simulink model "Controller"  (R2025a)
settings: Solver=FixedStepAuto  StartTime=0.0  StopTime=0.5  FixedStep=1e-6  RelTol=1e-3
undefined symbols (not defined in the file): Bit_1, Bit_2, Bit_3, Bit_4, Bit_5, Bit_6, Bit_7, Bit_8
libraries: simulink_extras x42, fl_lib x33, nesl_utility x17, simulink x4, dspsigops x2
(part 1 of 3)
settings Model: PacingRate=0.002500  Creator=Erys  LastModifiedBy=Erys
settings SolverCC: AllowMultiTaskInputOutput=on

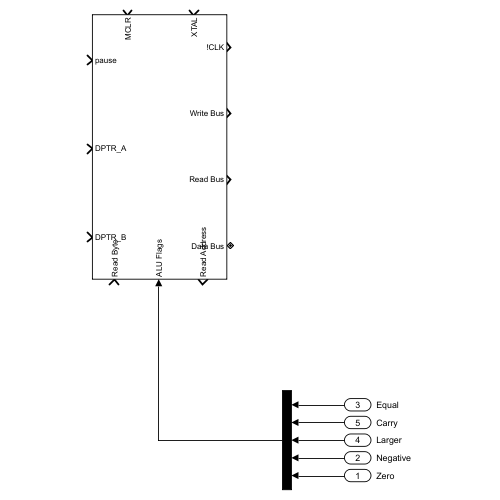
[thumbnail: Simulink's stored preview of the top-level diagram]
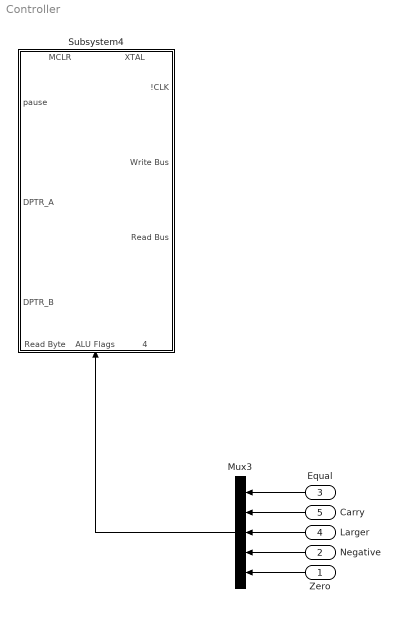
== system Controller ==
  Zero : Inport
  Negative : Inport  Port=2
  Equal : Inport  Port=3
  Larger : Inport  Port=4
  Carry : Inport  Port=5
  Mux3 : Mux  Inputs=5
  Subsystem4 : Subsystem
      settings: PortSchema="{\"entries\":[{\"content\":{\"sides\":[{\"content\":{\"connectorIds\":[\"In1\",\"In2\",\"In3\"]},\"type\":\"ConnectorPlacement.EquallySpacedRectSide\",\"uuid\":\"d5e2a106-9af6-429b-a75d-9517a76ca7ea\"},{\"content\":{\"connectorIds\":[\"Out1\",\"Out2\",\"Out3\",\"RConn1\"],\"side\":\"RIGHT\"},\"type\":\"ConnectorPlacement.EquallySpacedRectSide\",\"uuid\":\"6877b27f-1be8-45b2-a02e-770da90fb244\"},{\"content\":{\"connectorIds\":[\"In4\",\"In5\"],\"side\":\"TOP\"},\"type\":\"ConnectorPlacement.EquallySpacedRectSide\",\"uuid\":\"b2c1f94a-cab7-4390-a39c-f82c22ddd5ce\"},{\"content\":{\"connectorIds\":[\"In6\",\"In7\",\"Out4\"],\"side\":\"BOTTOM\"},\"type\":\"ConnectorPlacement.EquallySpacedRectSide\",\"uuid\":\"902a6980-cbbd-4700-8659-46292e270521\"}]},\"type\":\"ConnectorPlacement.EquallySpacedConnector\",\"uuid\":\"c8caef69-ab90-47f5-9596-0f6f8fcd412d\"}],\"packageUris\":[\"http://schema.mathworks.com/mf0/Connector/R2020b\"],\"version\":\"1.0\"}"
  wires:
  Larger/1 -> Mux3/3
  Zero/1 -> Mux3/5
  Negative/1 -> Mux3/4
  Equal/1 -> Mux3/1
  Carry/1 -> Mux3/2
  Mux3/1 -> Subsystem4/7(ALU Flags)

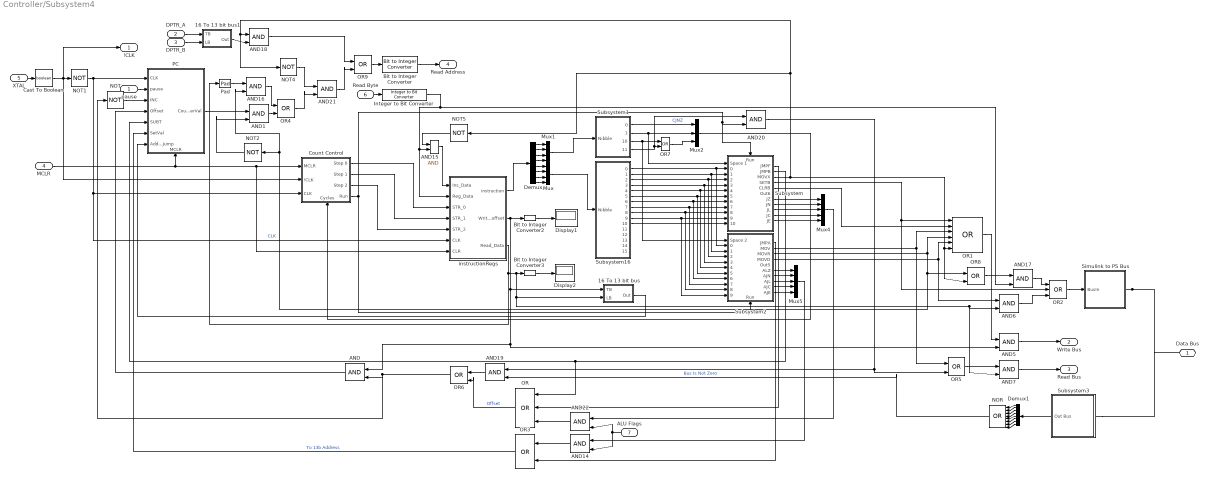
== system Controller/Subsystem4 ==
  pause : Inport
  DPTR_A : Inport  Port=2
  DPTR_B : Inport  Port=3
  MCLR : Inport  Port=4
  XTAL : Inport  Port=5
  Read Byte : Inport  Port=6
  ALU Flags : Inport  Port=7
  16 To 13 bit bus : Subsystem
  16 To 13 bit bus1 : Subsystem
  AND{,1,5..7,14..22} (14 alike) : Logic  IconShape=distinctive  AllPortsSameDT=off  OutDataTypeStr=boolean
  Bit to Integer Converter : simulink/Logic and Bit Operations/Bit to Integer Converter  nbits=13  bitOrder=MSB first  signedOutputValues=Unsigned  outDtype=Inherit via internal rule  outDtypeSigned=Inherit via internal rule
  Bit to Integer Converter2 : simulink/Logic and Bit Operations/Bit to Integer Converter  nbits=8  bitOrder=MSB first  signedOutputValues=Unsigned  outDtype=Inherit via internal rule  outDtypeSigned=Inherit via internal rule
  Bit to Integer Converter3 : simulink/Logic and Bit Operations/Bit to Integer Converter  nbits=8  bitOrder=MSB first  signedOutputValues=Unsigned  outDtype=Inherit via internal rule  outDtypeSigned=Inherit via internal rule
  Cast To Boolean : DataTypeConversion  OutDataTypeStr=boolean  SaturateOnIntegerOverflow=off  RndMeth=Floor
  Count Control : Subsystem
      settings: PortSchema="{\"entries\":[{\"content\":{\"sides\":[{\"content\":{\"connectorIds\":[\"In1\",\"In2\",\"In3\"]},\"type\":\"ConnectorPlacement.EquallySpacedRectSide\",\"uuid\":\"2946c837-3e9e-4d6d-a79b-eeee00653dec\"},{\"content\":{\"connectorIds\":[\"Out1\",\"Out2\",\"Out3\",\"Out4\"],\"side\":\"RIGHT\"},\"type\":\"ConnectorPlacement.EquallySpacedRectSide\",\"uuid\":\"31741f8e-3a86-46f4-9b5c-128a6668da37\"},{\"content\":{\"side\":\"TOP\"},\"type\":\"ConnectorPlacement.EquallySpacedRectSide\",\"uuid\":\"d0cf1acd-e26c-4fb6-8ea6-e97418659fa2\"},{\"content\":{\"connectorIds\":[\"In4\"],\"side\":\"BOTTOM\"},\"type\":\"ConnectorPlacement.EquallySpacedRectSide\",\"uuid\":\"e969e3c0-96c1-4acf-855c-d1f83bd67524\"}]},\"type\":\"ConnectorPlacement.EquallySpacedConnector\",\"uuid\":\"6217865d-f245-4d28-aa10-c01e5d783290\"}],\"packageUris\":[\"http://schema.mathworks.com/mf0/Connector/R2020b\"],\"version\":\"1.0\"}"
  Demux : Demux  Outputs=8
  Demux1 : Demux  Outputs=8
  Display1 : Display
  Display2 : Display
  Integer to Bit Converter : simulink/Logic and Bit Operations/Integer to Bit Converter  nbits=8  signedInputValues=Unsigned  bitOrder=MSB first  outDtype=Inherit via internal rule
  Mux : Mux
  Mux1 : Mux
  Mux2 : Mux  Inputs=3
  Mux4 : Mux  Inputs=5
  Mux5 : Mux  Inputs=5
  NOR : Logic  Operator=OR  Inputs=8  IconShape=distinctive  AllPortsSameDT=off  OutDataTypeStr=boolean
  NOT{,1..2,4..5} (5 alike) : Logic  Operator=NOT  IconShape=distinctive  AllPortsSameDT=off  OutDataTypeStr=boolean
  OR : Logic  Operator=OR  Inputs=3  IconShape=distinctive  AllPortsSameDT=off  OutDataTypeStr=boolean
  OR1 : Logic  Operator=OR  Inputs=6  IconShape=distinctive  AllPortsSameDT=off  OutDataTypeStr=boolean
  OR2 : Logic  Operator=OR  Inputs=3  IconShape=distinctive  AllPortsSameDT=off  OutDataTypeStr=boolean
  OR{3..9} (7 alike) : Logic  Operator=OR  IconShape=distinctive  AllPortsSameDT=off  OutDataTypeStr=boolean
  PC : Subsystem
      settings: PortSchema="{\"entries\":[{\"content\":{\"sides\":[{\"content\":{\"connectorIds\":[\"In1\",\"In2\",\"In3\",\"In4\",\"In5\",\"In6\",\"In7\"]},\"type\":\"ConnectorPlacement.EquallySpacedRectSide\",\"uuid\":\"447360f6-a9ef-4a9c-a715-cde64203432e\"},{\"content\":{\"connectorIds\":[\"Out1\"],\"side\":\"RIGHT\"},\"type\":\"ConnectorPlacement.EquallySpacedRectSide\",\"uuid\":\"8baf234e-02d5-44b8-81cb-8a80707fc347\"},{\"content\":{\"side\":\"TOP\"},\"type\":\"ConnectorPlacement.EquallySpacedRectSide\",\"uuid\":\"5f74c121-ef0f-4272-a153-104d7b2f50e7\"},{\"content\":{\"connectorIds\":[\"In8\"],\"side\":\"BOTTOM\"},\"type\":\"ConnectorPlacement.EquallySpacedRectSide\",\"uuid\":\"1b724eb9-c90a-41ee-9e1f-a1aa86a34cfc\"}]},\"type\":\"ConnectorPlacement.EquallySpacedConnector\",\"uuid\":\"abd2f1ff-4bc7-462e-9088-dc740170a27d\"}],\"packageUris\":[\"http://schema.mathworks.com/mf0/Connector/R2020b\"],\"version\":\"1.0\"}"
  Pad : dspsigops/Pad  padAlong=Columns  dimsToPad=1  valSrc=Specify via dialog  padVal=0  spec=Output size  padNumOutRowsSpecMethod=User-specified  numOutRows=13  padNumOutColsSpecMethod=User-specified  numOutCols=1  isVarDimsMode=off  padBeginning=0  padEnd=0  outSizeMode=User-specified  outSize=1  padSigAt=Beginning  trunc_flag=None  roundingMode=Floor  overflowMode=off  truncOrWrapMode=Truncate  wrap_flag=None
  Simulink to PS Bus : Subsystem
  Subsystem : Subsystem
      settings: PortSchema="{\"entries\":[{\"content\":{\"sides\":[{\"content\":{\"connectorIds\":[\"In1\",\"In2\",\"In3\",\"In4\",\"In5\",\"In6\",\"In7\",\"In8\",\"In9\",\"In10\",\"In11\",\"In12\"]},\"type\":\"ConnectorPlacement.EquallySpacedRectSide\",\"uuid\":\"cfbb32f0-f26b-4c66-8bd2-b70029f88bb0\"},{\"content\":{\"connectorIds\":[\"Out1\",\"Out2\",\"Out3\",\"Out4\",\"Out5\",\"Out6\",\"Out7\",\"Out8\",\"Out9\",\"Out10\",\"Out11\"],\"side\":\"RIGHT\"},\"type\":\"ConnectorPlacement.EquallySpacedRectSide\",\"uuid\":\"98f5ba87-6b95-4dd6-a355-88798db6b2fd\"},{\"content\":{\"connectorIds\":[\"In13\"],\"side\":\"TOP\"},\"type\":\"ConnectorPlacement.EquallySpacedRectSide\",\"uuid\":\"0d46a759-70c5-4c59-bf81-538ef6837c1f\"}]},\"type\":\"ConnectorPlacement.EquallySpacedConnector\",\"uuid\":\"e16d022d-bc87-42d5-a95e-dac1e9efe00b\"}],\"packageUris\":[\"http://schema.mathworks.com/mf0/Connector/R2020b\"],\"version\":\"1.0\"}"
  Subsystem1 : Subsystem
  Subsystem16 : Subsystem
  Subsystem2 : Subsystem
      settings: PortSchema="{\"entries\":[{\"content\":{\"sides\":[{\"content\":{\"connectorIds\":[\"In1\",\"In2\",\"In3\",\"In4\",\"In5\",\"In6\",\"In7\",\"In8\",\"In9\",\"In10\",\"In11\"]},\"type\":\"ConnectorPlacement.EquallySpacedRectSide\",\"uuid\":\"b0b83ebf-b15c-48e6-90da-0c85466b0112\"},{\"content\":{\"connectorIds\":[\"Out1\",\"Out2\",\"Out3\",\"Out4\",\"Out5\",\"Out6\",\"Out7\",\"Out8\",\"Out9\",\"Out10\"],\"side\":\"RIGHT\"},\"type\":\"ConnectorPlacement.EquallySpacedRectSide\",\"uuid\":\"3e9a574c-c2fc-44d4-b6d6-2fd6d79cf320\"},{\"content\":{\"side\":\"TOP\"},\"type\":\"ConnectorPlacement.EquallySpacedRectSide\",\"uuid\":\"d0111dce-9a98-4fcc-8b1f-a07207ba465c\"},{\"content\":{\"connectorIds\":[\"In12\"],\"side\":\"BOTTOM\"},\"type\":\"ConnectorPlacement.EquallySpacedRectSide\",\"uuid\":\"f4ec0d33-710b-4536-80bf-b2ccdd599d6b\"}]},\"type\":\"ConnectorPlacement.EquallySpacedConnector\",\"uuid\":\"77566f56-f460-4ec7-92f0-67352915e372\"}],\"packageUris\":[\"http://schema.mathworks.com/mf0/Connector/R2020b\"],\"version\":\"1.0\"}"
  Subsystem3 : Subsystem
  instructionRegs : Subsystem
  Data Bus : PMIOPort  Side=Right
  !CLK : Outport
  Write Bus : Outport  Port=2
  Read Bus : Outport  Port=3
  Read Address : Outport  Port=4
  wires:
  NOT/1 -> PC/3(INC)
  Mux/1 -> Subsystem16/1(Nibble)
  Subsystem/7(JZ) -> Mux4/1
  Subsystem/8(JN) -> Mux4/2
  Subsystem2/4(MOVD) -> AND6/1, OR1/5
  Subsystem2/1(JMPA) -> OR3/2
  MCLR/1 -> Count Control/1(MCLR), instructionRegs/7(CLR), PC/8(MCLR)
  Subsystem16/7(6) -> Subsystem2/8(6), Subsystem/8(6)
  Subsystem2/3(MOVR) -> AND16/2, NOT2/1, OR8/1, OR1/4
  Subsystem16/1(0) -> Subsystem/2(0), Subsystem2/2(0)
  Mux2/1 -> Count Control/4(Cycles)
  Subsystem16/8(7) -> Subsystem2/9(7), Subsystem/9(7)
  OR4/1 -> AND21/2
  AND5/1 -> Write Bus/1
  Subsystem/9(JL) -> Mux4/3
  Bit to Integer Converter3/1 -> Display2/1
  Demux/4 -> Mux1/4
  Subsystem16/4(3) -> Subsystem2/5(3), Subsystem/5(3)
  Subsystem/2(JMPB) -> OR/1, PC/5(SUBT)
  Subsystem/1(JMPF) -> OR/2
  Subsystem16/10(9) -> Subsystem2/11(9), Subsystem/11(9)
  Subsystem16/3(2) -> Subsystem2/4(2), Subsystem/4(2)
  OR/1 -> OR6/2  "Offset"
  AND7/1 -> Read Bus/1
  Subsystem/4(SETB) -> OR2/2, OR1/1
  Count Control/4(Run) -> AND20/2, Subsystem/13(Run), Subsystem2/12(Run)
  AND17/1 -> OR2/1
  Demux/6 -> Mux/2
  Demux/8 -> Mux/4
  Bit to Integer Converter2/1 -> Display1/1
  OR2/1 -> Simulink to PS Bus/1(BusIn)
  Demux/7 -> Mux/3
  Cast To Boolean/1 -> !CLK/1, Count Control/2(!CLK), NOT1/1
  Demux/3 -> Mux1/3
  Read Byte/1 -> Integer to Bit Converter/1
  Mux1/1 -> Subsystem1/1(Nibble)
  Subsystem16/9(8) -> Subsystem2/10(8), Subsystem/10(8)
  Subsystem16/6(5) -> Subsystem2/7(5), Subsystem/7(5)
  Bit to Integer Converter/1 -> Read Address/1
  Subsystem16/2(1) -> Subsystem/3(1), Subsystem2/3(1)
  Subsystem1/1(0) -> Mux2/1
  Subsystem2/2(MOV) -> OR5/1, OR1/3
  NOT1/1 -> instructionRegs/6(CLK), Count Control/3(CLK), PC/1(CLK)  "CLK"
  Integer to Bit Converter/1 -> instructionRegs/2(Reg_Data), AND15/2, AND17/2
  XTAL/1 -> Cast To Boolean/1
  AND16/1 -> OR4/1
  AND/1 -> PC/4(Offset)
  Subsystem16/11(10) -> Subsystem/12(10)
  Subsystem1/2(1) -> Mux2/2, Subsystem/1(Space 1)
  Subsystem/5(CLRB) -> OR1/2
  Demux/2 -> Mux1/2
  Demux/1 -> Mux1/1
  Subsystem16/5(4) -> Subsystem2/6(4), Subsystem/6(4)
  Subsystem1/3(10) -> OR7/1, Subsystem2/1(Space 2)
  OR1/1 -> AND5/1
  Demux/5 -> Mux/1
  OR5/1 -> AND7/1
  NOR/1 -> AND19/2  "Bus Is Not Zero"
  OR3/1 -> PC/6(SetVal)  "To 13b Address"
  PC/1(CounterVal) -> AND1/1
  AND1/1 -> OR4/2
  16 To 13 bit bus/1(Out) -> PC/7(AddressJump)
  Subsystem/10(JC) -> Mux4/4
  Demux1/2 -> NOR/2
  Subsystem/11(JE) -> Mux4/5
  Demux1/1 -> NOR/1
  AND14/1 -> OR3/1
  AND6/1 -> OR2/3
  NOT2/1 -> AND1/2
  Demux1/3 -> NOR/3
  Demux1/4 -> NOR/4
  Demux1/5 -> NOR/5
  Demux1/7 -> NOR/7
  Demux1/8 -> NOR/8
  Demux1/6 -> NOR/6
  Subsystem/3(MOVX) -> NOT5/1, NOT4/1, AND18/1, OR1/6, OR8/2
  pause/1 -> PC/2(pause)
  Subsystem1/4(11) -> AND20/1, OR7/2  "CJNZ"
  OR7/1 -> Mux2/3
  AND20/1 -> AND19/1, OR5/2
  OR6/1 -> NOT/1, AND/2
  AND19/1 -> OR6/1
  Subsystem3/1(Out Bus) -> Demux1/1
  16 To 13 bit bus1/1(Out) -> AND18/2
  DPTR_B/1 -> 16 To 13 bit bus1/2(LB)
  DPTR_A/1 -> 16 To 13 bit bus1/1(TB)
  Pad/1 -> AND16/1
  OR8/1 -> AND17/1
  NOT4/1 -> AND21/1
  AND21/1 -> OR9/2
  AND18/1 -> OR9/1
  OR9/1 -> Bit to Integer Converter/1
  NOT5/1 -> AND15/1
  instructionRegs/2(Write_offset) -> 16 To 13 bit bus/1(TB), AND/1, AND5/2, Bit to Integer Converter2/1
  instructionRegs/3(Read_Data) -> AND7/2, AND6/2, 16 To 13 bit bus/2(LB), Bit to Integer Converter3/1, Pad/1
  instructionRegs/1(instruction) -> Demux/1
  AND15/1 -> instructionRegs/1(Ins_Data)
  Count Control/1(Step 0) -> instructionRegs/3(STR_0)
  Count Control/2(Step 1) -> instructionRegs/4(STR_1)
  Count Control/3(Step 2) -> instructionRegs/5(STR_2)
  ALU Flags/1 -> AND22/2, AND14/2
  Mux4/1 -> AND22/1
  AND22/1 -> OR/3
  Subsystem2/10(AJE) -> Mux5/5
  Subsystem2/9(AJC) -> Mux5/4
  Subsystem2/8(AJL) -> Mux5/3
  Subsystem2/7(AJN) -> Mux5/2
  Subsystem2/6(ALZ) -> Mux5/1
  Mux5/1 -> AND14/1
  connections:
  Simulink to PS Bus/RConn1 -- Subsystem3/LConn1 -- Data Bus/RConn1

== system Controller/Subsystem4/16 To 13 bit bus ==
  TB : Inport
  LB : Inport  Port=2
  Demux1 : Demux  Outputs=8
  Demux2 : Demux  Outputs=8
  Mux2 : Mux  Inputs=13
  Out : Outport
  wires:
  Demux2/5 -> Mux2/10
  Demux1/8 -> Mux2/5
  Demux2/1 -> Mux2/6
  Demux1/5 -> Mux2/2
  Demux2/6 -> Mux2/11
  Demux1/6 -> Mux2/3
  Demux1/7 -> Mux2/4
  Demux2/2 -> Mux2/7
  Demux2/3 -> Mux2/8
  Demux1/4 -> Mux2/1
  Demux2/8 -> Mux2/13
  Demux2/7 -> Mux2/12
  Demux2/4 -> Mux2/9
  TB/1 -> Demux1/1
  Mux2/1 -> Out/1
  LB/1 -> Demux2/1

== system Controller/Subsystem4/16 To 13 bit bus1 ==
  TB : Inport
  LB : Inport  Port=2
  Demux1 : Demux  Outputs=8
  Demux2 : Demux  Outputs=8
  Mux2 : Mux  Inputs=13
  Out : Outport
  wires:
  Demux2/5 -> Mux2/10
  Demux1/8 -> Mux2/5
  Demux2/1 -> Mux2/6
  Demux1/5 -> Mux2/2
  Demux2/6 -> Mux2/11
  Demux1/6 -> Mux2/3
  Demux1/7 -> Mux2/4
  Demux2/2 -> Mux2/7
  Demux2/3 -> Mux2/8
  Demux1/4 -> Mux2/1
  Demux2/8 -> Mux2/13
  Demux2/7 -> Mux2/12
  Demux2/4 -> Mux2/9
  TB/1 -> Demux1/1
  Mux2/1 -> Out/1
  LB/1 -> Demux2/1

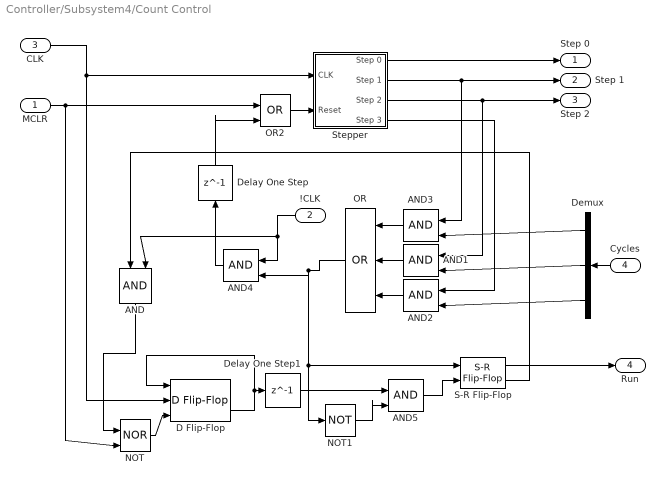
== system Controller/Subsystem4/Count Control ==
  MCLR : Inport
  !CLK : Inport  Port=2
  CLK : Inport  Port=3
  Cycles : Inport  Port=4
  AND{,1..5} (6 alike) : Logic  IconShape=distinctive  AllPortsSameDT=off  OutDataTypeStr=boolean
  D Flip-Flop : simulink_extras/Flip Flops/D Flip-Flop
  Delay One Step : Delay  DelayLength=1
  Delay One Step1 : Delay  DelayLength=1
  Demux : Demux  Outputs=3
  NOT : Logic  Operator=NOR  IconShape=distinctive  AllPortsSameDT=off  OutDataTypeStr=boolean
  NOT1 : Logic  Operator=NOT  IconShape=distinctive  AllPortsSameDT=off  OutDataTypeStr=boolean
  OR : Logic  Operator=OR  Inputs=3  IconShape=distinctive  AllPortsSameDT=off  OutDataTypeStr=boolean
  OR2 : Logic  Operator=OR  IconShape=distinctive  AllPortsSameDT=off  OutDataTypeStr=boolean
  S-R Flip-Flop : simulink_extras/Flip Flops/S-R Flip-Flop  initial_condition=0
  Stepper : Subsystem
  Step 0 : Outport
  Step 1 : Outport  Port=2
  Step 2 : Outport  Port=3
  Run : Outport  Port=4
  wires:
  NOT/1 -> D Flip-Flop/3
  CLK/1 -> D Flip-Flop/2, Stepper/1(CLK)
  Stepper/2(Step 1) -> Step 1/1, AND3/1
  Stepper/1(Step 0) -> Step 0/1
  AND2/1 -> OR/3
  D Flip-Flop/2 -> Delay One Step1/1, D Flip-Flop/1
  AND1/1 -> OR/2
  AND3/1 -> OR/1
  Delay One Step/1 -> OR2/2
  !CLK/1 -> AND4/1, AND/2
  AND4/1 -> Delay One Step/1
  Stepper/3(Step 2) -> Step 2/1, AND1/1
  OR/1 -> S-R Flip-Flop/1, NOT1/1, AND4/2
  OR2/1 -> Stepper/2(Reset)
  Stepper/4(Step 3) -> AND2/1
  Demux/1 -> AND3/2
  Demux/2 -> AND1/2
  Demux/3 -> AND2/2
  Cycles/1 -> Demux/1
  MCLR/1 -> NOT/2, OR2/1
  S-R Flip-Flop/1 -> Run/1
  AND5/1 -> S-R Flip-Flop/2
  NOT1/1 -> AND5/2
  AND/1 -> NOT/1
  S-R Flip-Flop/2 -> AND/1
  Delay One Step1/1 -> AND5/1

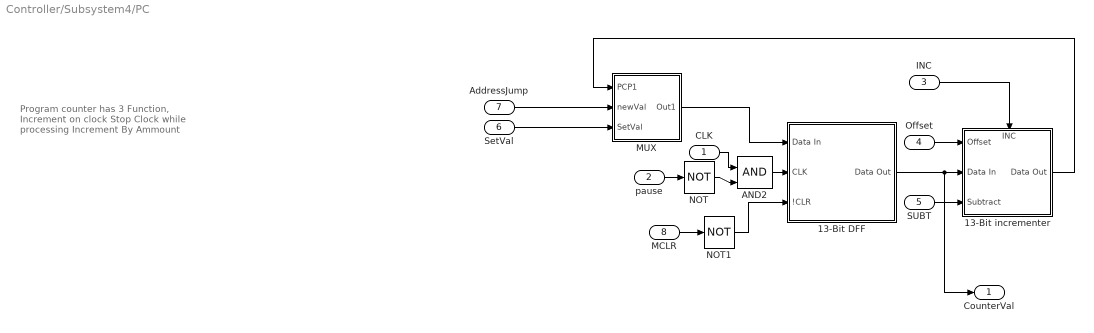
== system Controller/Subsystem4/PC ==
  note: Program counter has 3 Function,
      |
      | Increment on clock
      | Stop Clock while processing
      | Increment By Ammount
  CLK : Inport
  pause : Inport  Port=2
  INC : Inport  Port=3
  Offset : Inport  Port=4
  SUBT : Inport  Port=5
  SetVal : Inport  Port=6
  AddressJump : Inport  Port=7
  MCLR : Inport  Port=8
  "13-Bit DFF " : Subsystem
  13-Bit incrementer : Subsystem
      settings: PortSchema="{\"entries\":[{\"content\":{\"sides\":[{\"content\":{\"connectorIds\":[\"In1\",\"In2\",\"In3\"]},\"type\":\"ConnectorPlacement.EquallySpacedRectSide\",\"uuid\":\"739cec16-4094-4955-9615-f23c4a15ab23\"},{\"content\":{\"connectorIds\":[\"Out1\"],\"side\":\"RIGHT\"},\"type\":\"ConnectorPlacement.EquallySpacedRectSide\",\"uuid\":\"36202d39-d5af-435f-89aa-f53363edb9fe\"},{\"content\":{\"connectorIds\":[\"In4\"],\"side\":\"TOP\"},\"type\":\"ConnectorPlacement.EquallySpacedRectSide\",\"uuid\":\"08216fe9-0399-4cf5-9d97-18b54c3decd6\"}]},\"type\":\"ConnectorPlacement.EquallySpacedConnector\",\"uuid\":\"ce037f61-d800-42dc-bcb7-acda0bd23fde\"}],\"packageUris\":[\"http://schema.mathworks.com/mf0/Connector/R2020b\"],\"version\":\"1.0\"}"
  AND2 : Logic  IconShape=distinctive  AllPortsSameDT=off  OutDataTypeStr=boolean
  MUX : Subsystem
  NOT : Logic  Operator=NOT  IconShape=distinctive  AllPortsSameDT=off  OutDataTypeStr=boolean
  NOT1 : Logic  Operator=NOT  IconShape=distinctive  AllPortsSameDT=off  OutDataTypeStr=boolean
  CounterVal : Outport
  wires:
  CLK/1 -> AND2/1
  MCLR/1 -> NOT1/1
  "13-Bit DFF "/1(Data Out) -> CounterVal/1, 13-Bit incrementer/2(Data In)
  Offset/1 -> 13-Bit incrementer/1(Offset)
  INC/1 -> 13-Bit incrementer/4(INC)
  SUBT/1 -> 13-Bit incrementer/3(Subtract)
  NOT/1 -> AND2/2
  pause/1 -> NOT/1
  NOT1/1 -> "13-Bit DFF "/3(!CLR)
  AND2/1 -> "13-Bit DFF "/2(CLK)
  AddressJump/1 -> MUX/2(newVal)
  SetVal/1 -> MUX/3(SetVal)
  13-Bit incrementer/1(Data Out) -> MUX/1(PCP1)
  MUX/1(Out1) -> "13-Bit DFF "/1(Data In)

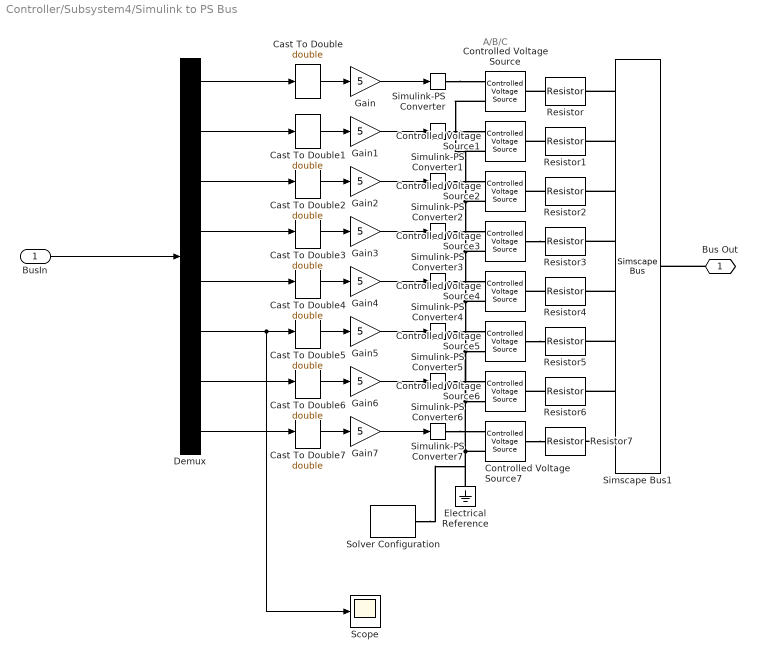
== system Controller/Subsystem4/Simulink to PS Bus ==
  note: A/B/C
  BusIn : Inport
  Cast To Double{,1..7} (8 alike) : DataTypeConversion  OutDataTypeStr=double  SaturateOnIntegerOverflow=off  RndMeth=Floor
  Controlled Voltage Source{,1..7} (8 alike) : fl_lib/Electrical/Electrical Sources/Controlled Voltage Source
  Demux : Demux  Outputs=8
  Electrical Reference : fl_lib/Electrical/Electrical Elements/Electrical Reference
  Gain{,1..7} (8 alike) : Gain  Gain=5
  Resistor{,1..7} (8 alike) : fl_lib/Electrical/Electrical Elements/Resistor  R=1 Ohm  i_specify=off  i_priority=None  i=0 A  i_nominal_specify=off  i_nominal_value=1  i_nominal_unit=A  v_specify=off  v_priority=None  v=0 V  v_nominal_specify=off  v_nominal_value=1  v_nominal_unit=V
  Scope : Scope
      settings: ActiveDisplayYMinimum=-0.125  ActiveDisplayYMaximum=1.125  DataLoggingVariableName=ScopeData2
  Simscape Bus1 : SimscapeBus  HierarchyStrings=Bit_8;Bit_7;Bit_6;Bit_5;Bit_4;Bit_3;Bit_2;Bit_1
  Simulink-PS Converter{,1..7} (8 alike) : nesl_utility/Simulink-PS Converter  PhysicalDomain=network_engine_domain  SubClassName=ps_input  LeftPortType=input  RightPortType=output  PseudoPeriodic=off  Frequencies=[]  NoiseDistribution=none  NoiseParameters=[]  Unit=1  AffineConversion=off  FilteringAndDerivatives=provide  SimscapeFilterOrder=1  InputFilterTimeConstant=0.001  UdotUserProvided=0
  Solver Configuration : nesl_utility/Solver Configuration  PhysicalDomain=network_engine_domain  SubClassName=solver  LeftPortType=input  RightPortType=generic  Tones=[]  Harmonics=[]  SimulateNoise=off  Profile=off  UseLocalSampling=off  EnableSwitchedLinearOptims=on  FrequencyDomain=off  UseCCode=off  RelTol=0.001  AbsTol=0.001  MinStep=1e-09  ToWorkspace=off  RevertToSquareIcSolve=off  NumHomotopyIterations=100  PhasorMode=off  PhasorModeNumHarmonics=1  ConsistencySolver=NEWTON_XTOL_AFTER_FTOL  IndexReductionMethod=DerivativeReplacement  DoDC=off  ResidualTolerance=1e-09  ConsistencyTolSource=GLOBAL  ConsistencyAbsTol=0.001  ConsistencyRelTol=0.001  ConsistencyTolFactor=0.001  UseLocalSolver=off  LocalSolverChoice=NE_BACKWARD_EULER_ADVANCER  ResolveIndetEquations=on  FunctionEvalNumThread=1  LocalSolverSampleTime=0.001  DoFixedCost=off  MaxNonlinIter=3  MaxModeIter=2  ComputeImpulses=off  ImpulseIterations=2  LinearAlgebra=auto  LinearAlgebraNumThread=0  EquationFormulation=NE_TIME_EF  DelaysMemoryBudget=1024  AutomaticFiltering=on  FilteringTimeConstant=0.001  PartitionStorageMethod=AS_NEEDED  PartitionMemoryBudget=1024  PartitionMethod=ROBUST  MultibodyUseLocalSolver=off  MultibodyLocalSolverChoice=ODE1  MultibodyLocalSolverSampleTime=0.001
  Bus Out : PMIOPort  Side=Right
  wires:
  BusIn/1 -> Demux/1
  Demux/5 -> Cast To Double4/1
  Cast To Double5/1 -> Gain5/1
  Cast To Double6/1 -> Gain6/1
  Cast To Double7/1 -> Gain7/1
  Gain/1 -> Simulink-PS Converter/1
  Demux/2 -> Cast To Double1/1
  Demux/4 -> Cast To Double3/1
  Gain5/1 -> Simulink-PS Converter5/1
  Gain4/1 -> Simulink-PS Converter4/1
  Gain2/1 -> Simulink-PS Converter2/1
  Cast To Double2/1 -> Gain2/1
  Cast To Double4/1 -> Gain4/1
  Gain6/1 -> Simulink-PS Converter6/1
  Cast To Double3/1 -> Gain3/1
  Cast To Double/1 -> Gain/1
  Cast To Double1/1 -> Gain1/1
  Demux/7 -> Cast To Double6/1
  Demux/1 -> Cast To Double/1
  Gain3/1 -> Simulink-PS Converter3/1
  Demux/6 -> Scope/1, Cast To Double5/1
  Gain7/1 -> Simulink-PS Converter7/1
  Demux/8 -> Cast To Double7/1
  Demux/3 -> Cast To Double2/1
  Gain1/1 -> Simulink-PS Converter1/1
  connections:
  Controlled Voltage Source2/RConn2 -- Controlled Voltage Source/RConn2 -- Controlled Voltage Source1/RConn2 -- Controlled Voltage Source5/RConn2 -- Solver Configuration/RConn1 -- Electrical Reference/LConn1 -- Controlled Voltage Source7/RConn2 -- Controlled Voltage Source6/RConn2 -- Controlled Voltage Source4/RConn2 -- Controlled Voltage Source3/RConn2
  Simscape Bus1/LConn7 -- Resistor6/RConn1
  Simscape Bus1/LConn5 -- Resistor4/RConn1
  Simscape Bus1/LConn8 -- Resistor7/RConn1
  Simulink-PS Converter5/RConn1 -- Controlled Voltage Source5/RConn1
  Simulink-PS Converter4/RConn1 -- Controlled Voltage Source4/RConn1
  Simulink-PS Converter6/RConn1 -- Controlled Voltage Source6/RConn1
  Simulink-PS Converter/RConn1 -- Controlled Voltage Source/RConn1
  Simulink-PS Converter1/RConn1 -- Controlled Voltage Source1/RConn1
  Simscape Bus1/LConn4 -- Resistor3/RConn1
  Controlled Voltage Source5/LConn1 -- Resistor5/LConn1
  Simulink-PS Converter7/RConn1 -- Controlled Voltage Source7/RConn1
  Simulink-PS Converter3/RConn1 -- Controlled Voltage Source3/RConn1
  Simscape Bus1/LConn2 -- Resistor1/RConn1
  Simulink-PS Converter2/RConn1 -- Controlled Voltage Source2/RConn1
  Resistor2/LConn1 -- Controlled Voltage Source2/LConn1
  Resistor/LConn1 -- Controlled Voltage Source/LConn1
  Simscape Bus1/LConn1 -- Resistor/RConn1
  Resistor1/LConn1 -- Controlled Voltage Source1/LConn1
  Simscape Bus1/LConn3 -- Resistor2/RConn1
  Controlled Voltage Source3/LConn1 -- Resistor3/LConn1
  Resistor4/LConn1 -- Controlled Voltage Source4/LConn1
  Simscape Bus1/LConn6 -- Resistor5/RConn1
  Resistor6/LConn1 -- Controlled Voltage Source6/LConn1
  Controlled Voltage Source7/LConn1 -- Resistor7/LConn1
  Bus Out/RConn1 -- Simscape Bus1/RConn1

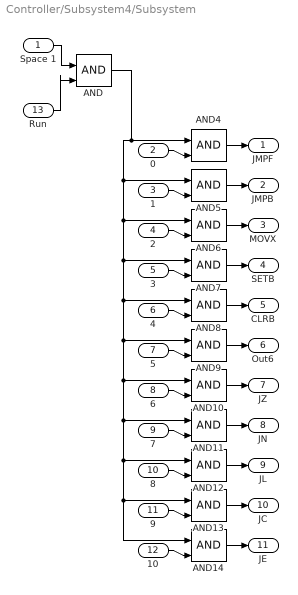
== system Controller/Subsystem4/Subsystem ==
  Space 1 : Inport
  0 : Inport  Port=2
  1 : Inport  Port=3
  2 : Inport  Port=4
  3 : Inport  Port=5
  4 : Inport  Port=6
  5 : Inport  Port=7
  6 : Inport  Port=8
  7 : Inport  Port=9
  8 : Inport  Port=10
  9 : Inport  Port=11
  10 : Inport  Port=12
  Run : Inport  Port=13
  AND{,4..14} (12 alike) : Logic  IconShape=distinctive  AllPortsSameDT=off  OutDataTypeStr=boolean
  JMPF : Outport
  JMPB : Outport  Port=2
  MOVX : Outport  Port=3
  SETB : Outport  Port=4
  CLRB : Outport  Port=5
  Out6 : Outport  Port=6
  JZ : Outport  Port=7
  JN : Outport  Port=8
  JL : Outport  Port=9
  JC : Outport  Port=10
  JE : Outport  Port=11
  wires:
  AND13/1 -> JC/1
  AND/1 -> AND14/1, AND13/1, AND12/1, AND11/1, AND10/1, AND9/1, AND8/1, AND7/1, AND6/1, AND5/1, AND4/1
  6/1 -> AND10/2
  AND12/1 -> JL/1
  AND14/1 -> JE/1
  0/1 -> AND4/2
  9/1 -> AND13/2
  AND10/1 -> JZ/1
  1/1 -> AND5/2
  7/1 -> AND11/2
  8/1 -> AND12/2
  AND6/1 -> MOVX/1
  2/1 -> AND6/2
  5/1 -> AND9/2
  4/1 -> AND8/2
  AND5/1 -> JMPB/1
  3/1 -> AND7/2
  AND8/1 -> CLRB/1
  AND11/1 -> JN/1
  AND4/1 -> JMPF/1
  AND7/1 -> SETB/1
  AND9/1 -> Out6/1
  10/1 -> AND14/2
  Space 1/1 -> AND/1
  Run/1 -> AND/2

== system Controller/Subsystem4/Subsystem1 ==
  Nibble : Inport
  AND{,1..3} (4 alike) : Logic  IconShape=distinctive  AllPortsSameDT=off  OutDataTypeStr=boolean
  Demux : Demux
  NOT2 : Logic  Operator=NOT  IconShape=distinctive  AllPortsSameDT=off  OutDataTypeStr=boolean
  NOT3 : Logic  Operator=NOT  IconShape=distinctive  AllPortsSameDT=off  OutDataTypeStr=boolean
  0 : Outport
  1 : Outport  Port=2
  10 : Outport  Port=3
  11 : Outport  Port=4
  wires:
  Nibble/1 -> Demux/1
  Demux/4 -> AND1/2, AND3/2, NOT3/1
  Demux/3 -> AND2/1, AND3/1, NOT2/1
  NOT2/1 -> AND1/1, AND/1
  NOT3/1 -> AND2/2, AND/2
  AND3/1 -> 11/1
  AND2/1 -> 10/1
  AND/1 -> 0/1
  AND1/1 -> 1/1

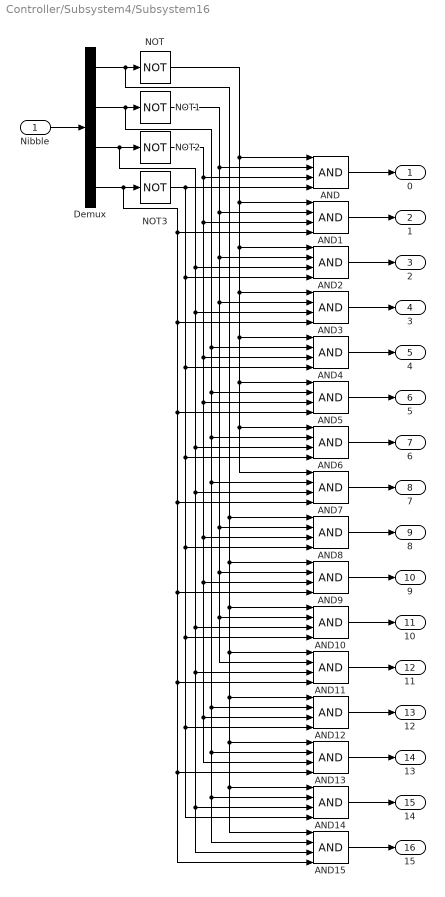
== system Controller/Subsystem4/Subsystem16 ==
  Nibble : Inport
  AND{,1..15} (16 alike) : Logic  Inputs=4  IconShape=distinctive  AllPortsSameDT=off  OutDataTypeStr=boolean
  Demux : Demux
  NOT{,1..3} (4 alike) : Logic  Operator=NOT  IconShape=distinctive  AllPortsSameDT=off  OutDataTypeStr=boolean
  0 : Outport
  1 : Outport  Port=2
  2 : Outport  Port=3
  3 : Outport  Port=4
  4 : Outport  Port=5
  5 : Outport  Port=6
  6 : Outport  Port=7
  7 : Outport  Port=8
  8 : Outport  Port=9
  9 : Outport  Port=10
  10 : Outport  Port=11
  11 : Outport  Port=12
  12 : Outport  Port=13
  13 : Outport  Port=14
  14 : Outport  Port=15
  15 : Outport  Port=16
  wires:
  Nibble/1 -> Demux/1
  Demux/1 -> NOT/1, AND8/1, AND15/1, AND14/1, AND13/1, AND12/1, AND11/1, AND10/1, AND9/1
  Demux/4 -> AND5/4, AND7/4, AND9/4, AND11/4, AND13/4, AND15/4, AND3/4, AND1/4, NOT3/1
  Demux/3 -> AND15/3, AND14/3, AND11/3, AND10/3, AND7/3, AND6/3, AND3/3, AND2/3, NOT2/1
  Demux/2 -> AND15/2, AND14/2, AND13/2, AND12/2, AND7/2, AND6/2, AND5/2, AND4/2, NOT1/1
  NOT/1 -> AND/1, AND7/1, AND6/1, AND5/1, AND4/1, AND3/1, AND2/1, AND1/1
  NOT1/1 -> AND/2, AND3/2, AND11/2, AND10/2, AND9/2, AND8/2, AND2/2, AND1/2
  NOT2/1 -> AND13/3, AND12/3, AND9/3, AND8/3, AND5/3, AND4/3, AND1/3, AND/3
  NOT3/1 -> AND14/4, AND12/4, AND10/4, AND8/4, AND6/4, AND4/4, AND2/4, AND/4
  AND15/1 -> 15/1
  AND14/1 -> 14/1
  AND13/1 -> 13/1
  AND12/1 -> 12/1
  AND11/1 -> 11/1
  AND10/1 -> 10/1
  AND9/1 -> 9/1
  AND8/1 -> 8/1
  AND7/1 -> 7/1
  AND6/1 -> 6/1
  AND5/1 -> 5/1
  AND4/1 -> 4/1
  AND3/1 -> 3/1
  AND2/1 -> 2/1
  AND/1 -> 0/1
  AND1/1 -> 1/1

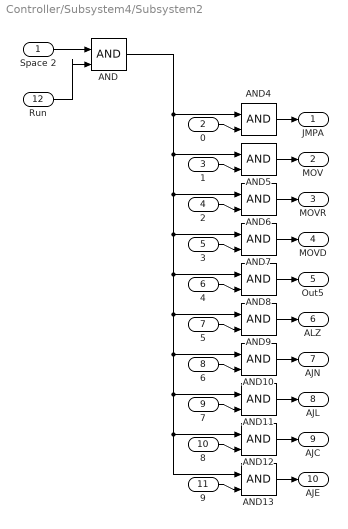
== system Controller/Subsystem4/Subsystem2 ==
  Space 2 : Inport
  0 : Inport  Port=2
  1 : Inport  Port=3
  2 : Inport  Port=4
  3 : Inport  Port=5
  4 : Inport  Port=6
  5 : Inport  Port=7
  6 : Inport  Port=8
  7 : Inport  Port=9
  8 : Inport  Port=10
  9 : Inport  Port=11
  Run : Inport  Port=12
  AND{,4..13} (11 alike) : Logic  IconShape=distinctive  AllPortsSameDT=off  OutDataTypeStr=boolean
  JMPA : Outport
  MOV : Outport  Port=2
  MOVR : Outport  Port=3
  MOVD : Outport  Port=4
  Out5 : Outport  Port=5
  ALZ : Outport  Port=6
  AJN : Outport  Port=7
  AJL : Outport  Port=8
  AJC : Outport  Port=9
  AJE : Outport  Port=10
  wires:
  AND13/1 -> AJE/1
  AND/1 -> AND13/1, AND12/1, AND11/1, AND10/1, AND9/1, AND8/1, AND7/1, AND6/1, AND5/1, AND4/1
  6/1 -> AND10/2
  AND12/1 -> AJC/1
  0/1 -> AND4/2
  9/1 -> AND13/2
  AND10/1 -> AJN/1
  1/1 -> AND5/2
  7/1 -> AND11/2
  8/1 -> AND12/2
  AND6/1 -> MOVR/1
  2/1 -> AND6/2
  5/1 -> AND9/2
  4/1 -> AND8/2
  AND5/1 -> MOV/1
  3/1 -> AND7/2
  AND8/1 -> Out5/1
  AND11/1 -> AJL/1
  AND4/1 -> JMPA/1
  AND7/1 -> MOVD/1
  AND9/1 -> ALZ/1
  Space 2/1 -> AND/1
  Run/1 -> AND/2

== system Controller/Subsystem4/Subsystem3 ==
  Mux : Mux  Inputs=8
  Simscape Bus2 : SimscapeBus  HierarchyStrings=Bit_8;Bit_7;Bit_6;Bit_5;Bit_4;Bit_3;Bit_2;Bit_1
  Subsystem1 : Subsystem
  Subsystem2 : Subsystem
  Subsystem3 : Subsystem
  Subsystem4 : Subsystem
  Subsystem5 : Subsystem
  Subsystem6 : Subsystem
  Subsystem7 : Subsystem
  Subsystem8 : Subsystem
  In Bus : PMIOPort  Side=Left
  Out Bus : Outport
  wires:
  Subsystem7/1(SIM) -> Mux/7
  Subsystem8/1(SIM) -> Mux/8
  Subsystem3/1(SIM) -> Mux/3
  Subsystem4/1(SIM) -> Mux/4
  Subsystem6/1(SIM) -> Mux/6
  Subsystem2/1(SIM) -> Mux/2
  Subsystem5/1(SIM) -> Mux/5
  Subsystem1/1(SIM) -> Mux/1
  Mux/1 -> Out Bus/1
  connections:
  Subsystem1/LConn1 -- Simscape Bus2/LConn1
  Simscape Bus2/LConn8 -- Subsystem8/LConn1
  Simscape Bus2/LConn5 -- Subsystem5/LConn1
  Simscape Bus2/LConn6 -- Subsystem6/LConn1
  Simscape Bus2/LConn7 -- Subsystem7/LConn1
  Simscape Bus2/LConn3 -- Subsystem3/LConn1
  Simscape Bus2/LConn4 -- Subsystem4/LConn1
  Simscape Bus2/LConn2 -- Subsystem2/LConn1
  In Bus/RConn1 -- Simscape Bus2/RConn1

== system Controller/Subsystem4/instructionRegs ==
  Ins_Data : Inport
  Reg_Data : Inport  Port=2
  STR_0 : Inport  Port=3
  STR_1 : Inport  Port=4
  STR_2 : Inport  Port=5
  CLK : Inport  Port=6
  CLR : Inport  Port=7
  Instruction : Subsystem
  Read/Data : Subsystem
  "Write/Offset " : Subsystem
  instruction : Outport
  Write_offset : Outport  Port=2
  Read_Data : Outport  Port=3
  wires:
  Ins_Data/1 -> Instruction/1(Ins_Data)
  STR_0/1 -> Instruction/2(Store)
  Instruction/1("Q Bus ") -> instruction/1
  STR_2/1 -> Read/Data/2(Store)
  CLK/1 -> Instruction/3(CLK), Read/Data/3(CLK), "Write/Offset "/3(CLK)
  Reg_Data/1 -> "Write/Offset "/1(Data bus), Read/Data/1(Data bus)
  CLR/1 -> "Write/Offset "/4(CLR), Read/Data/4(CLR), Instruction/4(CLR)
  "Write/Offset "/1("Q Bus ") -> Write_offset/1
  STR_1/1 -> "Write/Offset "/2(Store)
  Read/Data/1("Q Bus ") -> Read_Data/1

== system Controller/Subsystem4/Count Control/Stepper ==
  CLK : Inport
  Reset : Inport  Port=2
  Constant : Constant
  NOT : Logic  Operator=NOT  IconShape=distinctive  AllPortsSameDT=off  OutDataTypeStr=boolean
  Subsystem1 : Subsystem
      settings: PortSchema="{\"entries\":[{\"content\":{\"sides\":[{\"content\":{\"connectorIds\":[\"In1\",\"Out3\",\"In2\"]},\"type\":\"ConnectorPlacement.EquallySpacedRectSide\",\"uuid\":\"a2ffd4d4-cb1e-427b-87da-e82cfc528a9f\"},{\"content\":{\"connectorIds\":[\"Out1\",\"In4\",\"Out2\"],\"side\":\"RIGHT\"},\"type\":\"ConnectorPlacement.EquallySpacedRectSide\",\"uuid\":\"71314638-bff7-4a07-ab36-c1b86a64e6a5\"},{\"content\":{\"side\":\"TOP\"},\"type\":\"ConnectorPlacement.EquallySpacedRectSide\",\"uuid\":\"4ed90d18-bd24-4652-9ebf-70eb68655746\"},{\"content\":{\"connectorIds\":[\"In3\"],\"side\":\"BOTTOM\"},\"type\":\"ConnectorPlacement.EquallySpacedRectSide\",\"uuid\":\"b13ca18e-58ec-4b33-9e47-5b828845d5a6\"}]},\"type\":\"ConnectorPlacement.EquallySpacedConnector\",\"uuid\":\"af20c32a-17bf-45dc-90e2-7848574669b1\"}],\"packageUris\":[\"http://schema.mathworks.com/mf0/Connector/R2020b\"],\"version\":\"1.0\"}"
  Subsystem2 : Subsystem
      settings: PortSchema="{\"entries\":[{\"content\":{\"sides\":[{\"content\":{\"connectorIds\":[\"In1\",\"Out3\",\"In2\"]},\"type\":\"ConnectorPlacement.EquallySpacedRectSide\",\"uuid\":\"a2ffd4d4-cb1e-427b-87da-e82cfc528a9f\"},{\"content\":{\"connectorIds\":[\"Out1\",\"In4\",\"Out2\"],\"side\":\"RIGHT\"},\"type\":\"ConnectorPlacement.EquallySpacedRectSide\",\"uuid\":\"71314638-bff7-4a07-ab36-c1b86a64e6a5\"},{\"content\":{\"side\":\"TOP\"},\"type\":\"ConnectorPlacement.EquallySpacedRectSide\",\"uuid\":\"4ed90d18-bd24-4652-9ebf-70eb68655746\"},{\"content\":{\"connectorIds\":[\"In3\"],\"side\":\"BOTTOM\"},\"type\":\"ConnectorPlacement.EquallySpacedRectSide\",\"uuid\":\"b13ca18e-58ec-4b33-9e47-5b828845d5a6\"}]},\"type\":\"ConnectorPlacement.EquallySpacedConnector\",\"uuid\":\"af20c32a-17bf-45dc-90e2-7848574669b1\"}],\"packageUris\":[\"http://schema.mathworks.com/mf0/Connector/R2020b\"],\"version\":\"1.0\"}"
  Subsystem3 : Subsystem
      settings: PortSchema="{\"entries\":[{\"content\":{\"sides\":[{\"content\":{\"connectorIds\":[\"In1\",\"Out3\",\"In2\"]},\"type\":\"ConnectorPlacement.EquallySpacedRectSide\",\"uuid\":\"a2ffd4d4-cb1e-427b-87da-e82cfc528a9f\"},{\"content\":{\"connectorIds\":[\"Out1\",\"In4\",\"Out2\"],\"side\":\"RIGHT\"},\"type\":\"ConnectorPlacement.EquallySpacedRectSide\",\"uuid\":\"71314638-bff7-4a07-ab36-c1b86a64e6a5\"},{\"content\":{\"side\":\"TOP\"},\"type\":\"ConnectorPlacement.EquallySpacedRectSide\",\"uuid\":\"4ed90d18-bd24-4652-9ebf-70eb68655746\"},{\"content\":{\"connectorIds\":[\"In3\"],\"side\":\"BOTTOM\"},\"type\":\"ConnectorPlacement.EquallySpacedRectSide\",\"uuid\":\"b13ca18e-58ec-4b33-9e47-5b828845d5a6\"}]},\"type\":\"ConnectorPlacement.EquallySpacedConnector\",\"uuid\":\"af20c32a-17bf-45dc-90e2-7848574669b1\"}],\"packageUris\":[\"http://schema.mathworks.com/mf0/Connector/R2020b\"],\"version\":\"1.0\"}"
  Step 0 : Outport
  Step 1 : Outport  Port=2
  Step 2 : Outport  Port=3
  Step 3 : Outport  Port=4
  wires:
  CLK/1 -> Subsystem3/2(CLK), Subsystem1/2(CLK), Subsystem2/2(CLK)
  Constant/1 -> Subsystem2/1("Step_{n-1}")
  Subsystem2/1("Step_{n}") -> Step 1/1, Subsystem1/1("Step_{n-1}")
  Subsystem1/3("OR_{n}") -> Subsystem2/4("OR_{n+1}")
  Subsystem1/1("Step_{n}") -> Subsystem3/1("Step_{n-1}"), Step 2/1
  Subsystem3/3("OR_{n}") -> Subsystem1/4("OR_{n+1}")
  Subsystem3/1("Step_{n}") -> Step 3/1
  Subsystem2/2("!Step_{n}") -> Step 0/1
  NOT/1 -> Subsystem3/3(!CLR), Subsystem1/3(!CLR), Subsystem2/3(!CLR)
  Reset/1 -> NOT/1, Subsystem3/4("OR_{n+1}")

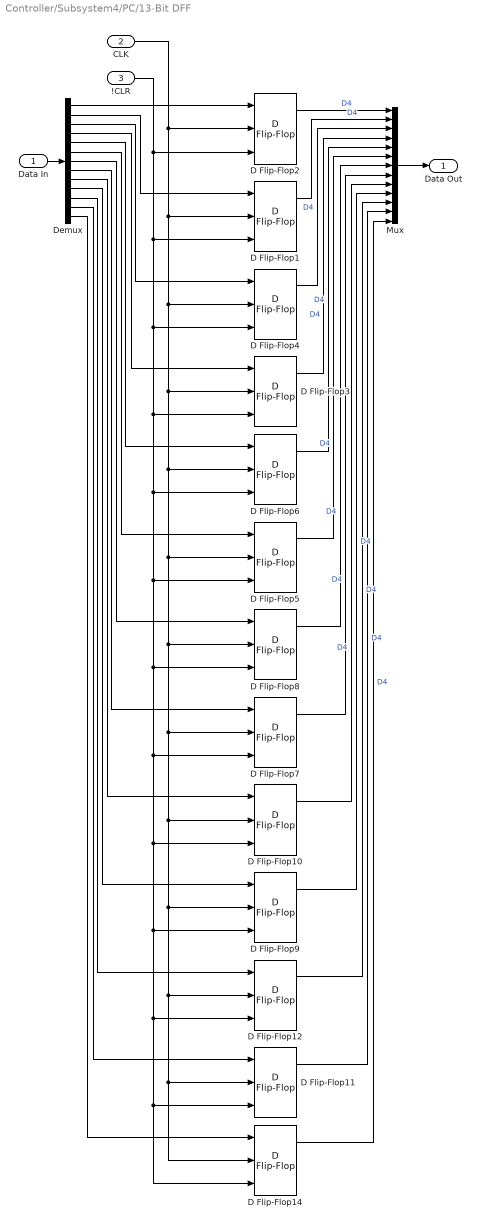
== system Controller/Subsystem4/PC/13-Bit DFF  ==
  Data In : Inport
  CLK : Inport  Port=2
  !CLR : Inport  Port=3
  D Flip-Flop{1..12,14} (13 alike) : simulink_extras/Flip Flops/D Flip-Flop
  Demux : Demux  Outputs=13
  Mux : Mux  Inputs=13
  Data Out : Outport
  wires:
  Data In/1 -> Demux/1
  Mux/1 -> Data Out/1
  !CLR/1 -> D Flip-Flop4/3, D Flip-Flop3/3, D Flip-Flop6/3, D Flip-Flop8/3, D Flip-Flop12/3, D Flip-Flop11/3, D Flip-Flop14/3, D Flip-Flop9/3, D Flip-Flop10/3, D Flip-Flop7/3, D Flip-Flop5/3, D Flip-Flop1/3, D Flip-Flop2/3
  CLK/1 -> D Flip-Flop1/2, D Flip-Flop6/2, D Flip-Flop5/2, D Flip-Flop8/2, D Flip-Flop9/2, D Flip-Flop14/2, D Flip-Flop11/2, D Flip-Flop12/2, D Flip-Flop10/2, D Flip-Flop7/2, D Flip-Flop3/2, D Flip-Flop4/2, D Flip-Flop2/2
  Demux/1 -> D Flip-Flop2/1
  Demux/2 -> D Flip-Flop1/1
  Demux/3 -> D Flip-Flop4/1
  Demux/4 -> D Flip-Flop3/1
  Demux/5 -> D Flip-Flop6/1
  Demux/6 -> D Flip-Flop5/1
  Demux/7 -> D Flip-Flop8/1
  Demux/8 -> D Flip-Flop7/1
  Demux/9 -> D Flip-Flop10/1
  Demux/10 -> D Flip-Flop9/1
  Demux/11 -> D Flip-Flop12/1
  Demux/12 -> D Flip-Flop11/1
  Demux/13 -> D Flip-Flop14/1
  D Flip-Flop2/1 -> Mux/1  "D4"
  D Flip-Flop1/1 -> Mux/2  "D4"
  D Flip-Flop4/1 -> Mux/3  "D4"
  D Flip-Flop3/1 -> Mux/4  "D4"
  D Flip-Flop6/1 -> Mux/5  "D4"
  D Flip-Flop5/1 -> Mux/6  "D4"
  D Flip-Flop8/1 -> Mux/7  "D4"
  D Flip-Flop7/1 -> Mux/8  "D4"
  D Flip-Flop10/1 -> Mux/9  "D4"
  D Flip-Flop9/1 -> Mux/10  "D4"
  D Flip-Flop12/1 -> Mux/11  "D4"
  D Flip-Flop11/1 -> Mux/12  "D4"
  D Flip-Flop14/1 -> Mux/13  "D4"

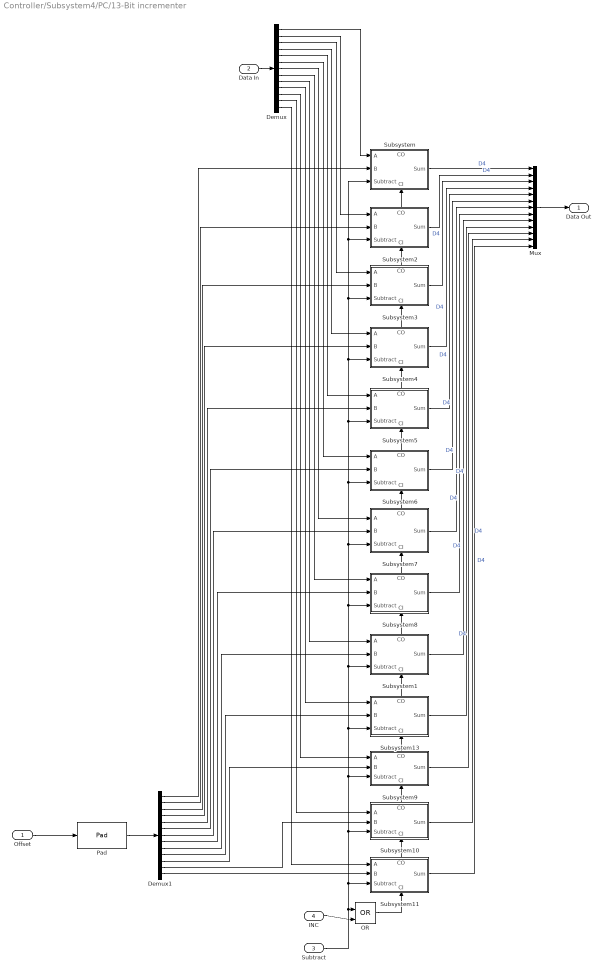
== system Controller/Subsystem4/PC/13-Bit incrementer ==
  Offset : Inport
  Data In : Inport  Port=2
  Subtract : Inport  Port=3
  INC : Inport  Port=4
  Demux : Demux  Outputs=13
  Demux1 : Demux  Outputs=13
  Mux : Mux  Inputs=13
  OR : Logic  Operator=OR  IconShape=distinctive  AllPortsSameDT=off  OutDataTypeStr=boolean
  Pad : dspsigops/Pad  padAlong=Columns  dimsToPad=1  valSrc=Specify via dialog  padVal=0  spec=Output size  padNumOutRowsSpecMethod=User-specified  numOutRows=13  padNumOutColsSpecMethod=User-specified  numOutCols=1  isVarDimsMode=off  padBeginning=0  padEnd=0  outSizeMode=User-specified  outSize=1  padSigAt=Beginning  trunc_flag=None  roundingMode=Floor  overflowMode=off  truncOrWrapMode=Truncate  wrap_flag=None
  Subsystem : Subsystem
      settings: PortSchema="{\"entries\":[{\"content\":{\"sides\":[{\"content\":{\"connectorIds\":[\"In1\",\"In2\",\"In3\"]},\"type\":\"ConnectorPlacement.EquallySpacedRectSide\",\"uuid\":\"3b61df12-5278-441c-99ea-cd13bbe6a5f0\"},{\"content\":{\"connectorIds\":[\"Out1\"],\"side\":\"RIGHT\"},\"type\":\"ConnectorPlacement.EquallySpacedRectSide\",\"uuid\":\"d74b7cc5-7b27-4e0f-8d84-952eb44d2cfa\"},{\"content\":{\"connectorIds\":[\"Out2\"],\"side\":\"TOP\"},\"type\":\"ConnectorPlacement.EquallySpacedRectSide\",\"uuid\":\"99314f25-b6d9-4ea5-a032-83307ae4bc34\"},{\"content\":{\"connectorIds\":[\"In4\"],\"side\":\"BOTTOM\"},\"type\":\"ConnectorPlacement.EquallySpacedRectSide\",\"uuid\":\"c9c43d88-8d1b-4564-af22-30722c8258ba\"}]},\"type\":\"ConnectorPlacement.EquallySpacedConnector\",\"uuid\":\"25cc7102-d96a-4215-b1b2-f44cf7e448cb\"}],\"packageUris\":[\"http://schema.mathworks.com/mf0/Connector/R2020b\"],\"version\":\"1.0\"}"
  Subsystem1 : Subsystem
      settings: PortSchema="{\"entries\":[{\"content\":{\"sides\":[{\"content\":{\"connectorIds\":[\"In1\",\"In2\",\"In3\"]},\"type\":\"ConnectorPlacement.EquallySpacedRectSide\",\"uuid\":\"3b61df12-5278-441c-99ea-cd13bbe6a5f0\"},{\"content\":{\"connectorIds\":[\"Out1\"],\"side\":\"RIGHT\"},\"type\":\"ConnectorPlacement.EquallySpacedRectSide\",\"uuid\":\"d74b7cc5-7b27-4e0f-8d84-952eb44d2cfa\"},{\"content\":{\"connectorIds\":[\"Out2\"],\"side\":\"TOP\"},\"type\":\"ConnectorPlacement.EquallySpacedRectSide\",\"uuid\":\"99314f25-b6d9-4ea5-a032-83307ae4bc34\"},{\"content\":{\"connectorIds\":[\"In4\"],\"side\":\"BOTTOM\"},\"type\":\"ConnectorPlacement.EquallySpacedRectSide\",\"uuid\":\"c9c43d88-8d1b-4564-af22-30722c8258ba\"}]},\"type\":\"ConnectorPlacement.EquallySpacedConnector\",\"uuid\":\"25cc7102-d96a-4215-b1b2-f44cf7e448cb\"}],\"packageUris\":[\"http://schema.mathworks.com/mf0/Connector/R2020b\"],\"version\":\"1.0\"}"
  Subsystem10 : Subsystem
      settings: PortSchema="{\"entries\":[{\"content\":{\"sides\":[{\"content\":{\"connectorIds\":[\"In1\",\"In2\",\"In3\"]},\"type\":\"ConnectorPlacement.EquallySpacedRectSide\",\"uuid\":\"3b61df12-5278-441c-99ea-cd13bbe6a5f0\"},{\"content\":{\"connectorIds\":[\"Out1\"],\"side\":\"RIGHT\"},\"type\":\"ConnectorPlacement.EquallySpacedRectSide\",\"uuid\":\"d74b7cc5-7b27-4e0f-8d84-952eb44d2cfa\"},{\"content\":{\"connectorIds\":[\"Out2\"],\"side\":\"TOP\"},\"type\":\"ConnectorPlacement.EquallySpacedRectSide\",\"uuid\":\"99314f25-b6d9-4ea5-a032-83307ae4bc34\"},{\"content\":{\"connectorIds\":[\"In4\"],\"side\":\"BOTTOM\"},\"type\":\"ConnectorPlacement.EquallySpacedRectSide\",\"uuid\":\"c9c43d88-8d1b-4564-af22-30722c8258ba\"}]},\"type\":\"ConnectorPlacement.EquallySpacedConnector\",\"uuid\":\"25cc7102-d96a-4215-b1b2-f44cf7e448cb\"}],\"packageUris\":[\"http://schema.mathworks.com/mf0/Connector/R2020b\"],\"version\":\"1.0\"}"
  Subsystem11 : Subsystem
      settings: PortSchema="{\"entries\":[{\"content\":{\"sides\":[{\"content\":{\"connectorIds\":[\"In1\",\"In2\",\"In3\"]},\"type\":\"ConnectorPlacement.EquallySpacedRectSide\",\"uuid\":\"3b61df12-5278-441c-99ea-cd13bbe6a5f0\"},{\"content\":{\"connectorIds\":[\"Out1\"],\"side\":\"RIGHT\"},\"type\":\"ConnectorPlacement.EquallySpacedRectSide\",\"uuid\":\"d74b7cc5-7b27-4e0f-8d84-952eb44d2cfa\"},{\"content\":{\"connectorIds\":[\"Out2\"],\"side\":\"TOP\"},\"type\":\"ConnectorPlacement.EquallySpacedRectSide\",\"uuid\":\"99314f25-b6d9-4ea5-a032-83307ae4bc34\"},{\"content\":{\"connectorIds\":[\"In4\"],\"side\":\"BOTTOM\"},\"type\":\"ConnectorPlacement.EquallySpacedRectSide\",\"uuid\":\"c9c43d88-8d1b-4564-af22-30722c8258ba\"}]},\"type\":\"ConnectorPlacement.EquallySpacedConnector\",\"uuid\":\"25cc7102-d96a-4215-b1b2-f44cf7e448cb\"}],\"packageUris\":[\"http://schema.mathworks.com/mf0/Connector/R2020b\"],\"version\":\"1.0\"}"
  Subsystem13 : Subsystem
      settings: PortSchema="{\"entries\":[{\"content\":{\"sides\":[{\"content\":{\"connectorIds\":[\"In1\",\"In2\",\"In3\"]},\"type\":\"ConnectorPlacement.EquallySpacedRectSide\",\"uuid\":\"3b61df12-5278-441c-99ea-cd13bbe6a5f0\"},{\"content\":{\"connectorIds\":[\"Out1\"],\"side\":\"RIGHT\"},\"type\":\"ConnectorPlacement.EquallySpacedRectSide\",\"uuid\":\"d74b7cc5-7b27-4e0f-8d84-952eb44d2cfa\"},{\"content\":{\"connectorIds\":[\"Out2\"],\"side\":\"TOP\"},\"type\":\"ConnectorPlacement.EquallySpacedRectSide\",\"uuid\":\"99314f25-b6d9-4ea5-a032-83307ae4bc34\"},{\"content\":{\"connectorIds\":[\"In4\"],\"side\":\"BOTTOM\"},\"type\":\"ConnectorPlacement.EquallySpacedRectSide\",\"uuid\":\"c9c43d88-8d1b-4564-af22-30722c8258ba\"}]},\"type\":\"ConnectorPlacement.EquallySpacedConnector\",\"uuid\":\"25cc7102-d96a-4215-b1b2-f44cf7e448cb\"}],\"packageUris\":[\"http://schema.mathworks.com/mf0/Connector/R2020b\"],\"version\":\"1.0\"}"
  Subsystem2 : Subsystem
      settings: PortSchema="{\"entries\":[{\"content\":{\"sides\":[{\"content\":{\"connectorIds\":[\"In1\",\"In2\",\"In3\"]},\"type\":\"ConnectorPlacement.EquallySpacedRectSide\",\"uuid\":\"3b61df12-5278-441c-99ea-cd13bbe6a5f0\"},{\"content\":{\"connectorIds\":[\"Out1\"],\"side\":\"RIGHT\"},\"type\":\"ConnectorPlacement.EquallySpacedRectSide\",\"uuid\":\"d74b7cc5-7b27-4e0f-8d84-952eb44d2cfa\"},{\"content\":{\"connectorIds\":[\"Out2\"],\"side\":\"TOP\"},\"type\":\"ConnectorPlacement.EquallySpacedRectSide\",\"uuid\":\"99314f25-b6d9-4ea5-a032-83307ae4bc34\"},{\"content\":{\"connectorIds\":[\"In4\"],\"side\":\"BOTTOM\"},\"type\":\"ConnectorPlacement.EquallySpacedRectSide\",\"uuid\":\"c9c43d88-8d1b-4564-af22-30722c8258ba\"}]},\"type\":\"ConnectorPlacement.EquallySpacedConnector\",\"uuid\":\"25cc7102-d96a-4215-b1b2-f44cf7e448cb\"}],\"packageUris\":[\"http://schema.mathworks.com/mf0/Connector/R2020b\"],\"version\":\"1.0\"}"
  Subsystem3 : Subsystem
      settings: PortSchema="{\"entries\":[{\"content\":{\"sides\":[{\"content\":{\"connectorIds\":[\"In1\",\"In2\",\"In3\"]},\"type\":\"ConnectorPlacement.EquallySpacedRectSide\",\"uuid\":\"3b61df12-5278-441c-99ea-cd13bbe6a5f0\"},{\"content\":{\"connectorIds\":[\"Out1\"],\"side\":\"RIGHT\"},\"type\":\"ConnectorPlacement.EquallySpacedRectSide\",\"uuid\":\"d74b7cc5-7b27-4e0f-8d84-952eb44d2cfa\"},{\"content\":{\"connectorIds\":[\"Out2\"],\"side\":\"TOP\"},\"type\":\"ConnectorPlacement.EquallySpacedRectSide\",\"uuid\":\"99314f25-b6d9-4ea5-a032-83307ae4bc34\"},{\"content\":{\"connectorIds\":[\"In4\"],\"side\":\"BOTTOM\"},\"type\":\"ConnectorPlacement.EquallySpacedRectSide\",\"uuid\":\"c9c43d88-8d1b-4564-af22-30722c8258ba\"}]},\"type\":\"ConnectorPlacement.EquallySpacedConnector\",\"uuid\":\"25cc7102-d96a-4215-b1b2-f44cf7e448cb\"}],\"packageUris\":[\"http://schema.mathworks.com/mf0/Connector/R2020b\"],\"version\":\"1.0\"}"
  Subsystem4 : Subsystem
      settings: PortSchema="{\"entries\":[{\"content\":{\"sides\":[{\"content\":{\"connectorIds\":[\"In1\",\"In2\",\"In3\"]},\"type\":\"ConnectorPlacement.EquallySpacedRectSide\",\"uuid\":\"3b61df12-5278-441c-99ea-cd13bbe6a5f0\"},{\"content\":{\"connectorIds\":[\"Out1\"],\"side\":\"RIGHT\"},\"type\":\"ConnectorPlacement.EquallySpacedRectSide\",\"uuid\":\"d74b7cc5-7b27-4e0f-8d84-952eb44d2cfa\"},{\"content\":{\"connectorIds\":[\"Out2\"],\"side\":\"TOP\"},\"type\":\"ConnectorPlacement.EquallySpacedRectSide\",\"uuid\":\"99314f25-b6d9-4ea5-a032-83307ae4bc34\"},{\"content\":{\"connectorIds\":[\"In4\"],\"side\":\"BOTTOM\"},\"type\":\"ConnectorPlacement.EquallySpacedRectSide\",\"uuid\":\"c9c43d88-8d1b-4564-af22-30722c8258ba\"}]},\"type\":\"ConnectorPlacement.EquallySpacedConnector\",\"uuid\":\"25cc7102-d96a-4215-b1b2-f44cf7e448cb\"}],\"packageUris\":[\"http://schema.mathworks.com/mf0/Connector/R2020b\"],\"version\":\"1.0\"}"
  Subsystem5 : Subsystem
      settings: PortSchema="{\"entries\":[{\"content\":{\"sides\":[{\"content\":{\"connectorIds\":[\"In1\",\"In2\",\"In3\"]},\"type\":\"ConnectorPlacement.EquallySpacedRectSide\",\"uuid\":\"3b61df12-5278-441c-99ea-cd13bbe6a5f0\"},{\"content\":{\"connectorIds\":[\"Out1\"],\"side\":\"RIGHT\"},\"type\":\"ConnectorPlacement.EquallySpacedRectSide\",\"uuid\":\"d74b7cc5-7b27-4e0f-8d84-952eb44d2cfa\"},{\"content\":{\"connectorIds\":[\"Out2\"],\"side\":\"TOP\"},\"type\":\"ConnectorPlacement.EquallySpacedRectSide\",\"uuid\":\"99314f25-b6d9-4ea5-a032-83307ae4bc34\"},{\"content\":{\"connectorIds\":[\"In4\"],\"side\":\"BOTTOM\"},\"type\":\"ConnectorPlacement.EquallySpacedRectSide\",\"uuid\":\"c9c43d88-8d1b-4564-af22-30722c8258ba\"}]},\"type\":\"ConnectorPlacement.EquallySpacedConnector\",\"uuid\":\"25cc7102-d96a-4215-b1b2-f44cf7e448cb\"}],\"packageUris\":[\"http://schema.mathworks.com/mf0/Connector/R2020b\"],\"version\":\"1.0\"}"
  Subsystem6 : Subsystem
      settings: PortSchema="{\"entries\":[{\"content\":{\"sides\":[{\"content\":{\"connectorIds\":[\"In1\",\"In2\",\"In3\"]},\"type\":\"ConnectorPlacement.EquallySpacedRectSide\",\"uuid\":\"3b61df12-5278-441c-99ea-cd13bbe6a5f0\"},{\"content\":{\"connectorIds\":[\"Out1\"],\"side\":\"RIGHT\"},\"type\":\"ConnectorPlacement.EquallySpacedRectSide\",\"uuid\":\"d74b7cc5-7b27-4e0f-8d84-952eb44d2cfa\"},{\"content\":{\"connectorIds\":[\"Out2\"],\"side\":\"TOP\"},\"type\":\"ConnectorPlacement.EquallySpacedRectSide\",\"uuid\":\"99314f25-b6d9-4ea5-a032-83307ae4bc34\"},{\"content\":{\"connectorIds\":[\"In4\"],\"side\":\"BOTTOM\"},\"type\":\"ConnectorPlacement.EquallySpacedRectSide\",\"uuid\":\"c9c43d88-8d1b-4564-af22-30722c8258ba\"}]},\"type\":\"ConnectorPlacement.EquallySpacedConnector\",\"uuid\":\"25cc7102-d96a-4215-b1b2-f44cf7e448cb\"}],\"packageUris\":[\"http://schema.mathworks.com/mf0/Connector/R2020b\"],\"version\":\"1.0\"}"
  Subsystem7 : Subsystem
      settings: PortSchema="{\"entries\":[{\"content\":{\"sides\":[{\"content\":{\"connectorIds\":[\"In1\",\"In2\",\"In3\"]},\"type\":\"ConnectorPlacement.EquallySpacedRectSide\",\"uuid\":\"3b61df12-5278-441c-99ea-cd13bbe6a5f0\"},{\"content\":{\"connectorIds\":[\"Out1\"],\"side\":\"RIGHT\"},\"type\":\"ConnectorPlacement.EquallySpacedRectSide\",\"uuid\":\"d74b7cc5-7b27-4e0f-8d84-952eb44d2cfa\"},{\"content\":{\"connectorIds\":[\"Out2\"],\"side\":\"TOP\"},\"type\":\"ConnectorPlacement.EquallySpacedRectSide\",\"uuid\":\"99314f25-b6d9-4ea5-a032-83307ae4bc34\"},{\"content\":{\"connectorIds\":[\"In4\"],\"side\":\"BOTTOM\"},\"type\":\"ConnectorPlacement.EquallySpacedRectSide\",\"uuid\":\"c9c43d88-8d1b-4564-af22-30722c8258ba\"}]},\"type\":\"ConnectorPlacement.EquallySpacedConnector\",\"uuid\":\"25cc7102-d96a-4215-b1b2-f44cf7e448cb\"}],\"packageUris\":[\"http://schema.mathworks.com/mf0/Connector/R2020b\"],\"version\":\"1.0\"}"
  Subsystem8 : Subsystem
      settings: PortSchema="{\"entries\":[{\"content\":{\"sides\":[{\"content\":{\"connectorIds\":[\"In1\",\"In2\",\"In3\"]},\"type\":\"ConnectorPlacement.EquallySpacedRectSide\",\"uuid\":\"3b61df12-5278-441c-99ea-cd13bbe6a5f0\"},{\"content\":{\"connectorIds\":[\"Out1\"],\"side\":\"RIGHT\"},\"type\":\"ConnectorPlacement.EquallySpacedRectSide\",\"uuid\":\"d74b7cc5-7b27-4e0f-8d84-952eb44d2cfa\"},{\"content\":{\"connectorIds\":[\"Out2\"],\"side\":\"TOP\"},\"type\":\"ConnectorPlacement.EquallySpacedRectSide\",\"uuid\":\"99314f25-b6d9-4ea5-a032-83307ae4bc34\"},{\"content\":{\"connectorIds\":[\"In4\"],\"side\":\"BOTTOM\"},\"type\":\"ConnectorPlacement.EquallySpacedRectSide\",\"uuid\":\"c9c43d88-8d1b-4564-af22-30722c8258ba\"}]},\"type\":\"ConnectorPlacement.EquallySpacedConnector\",\"uuid\":\"25cc7102-d96a-4215-b1b2-f44cf7e448cb\"}],\"packageUris\":[\"http://schema.mathworks.com/mf0/Connector/R2020b\"],\"version\":\"1.0\"}"
  Subsystem9 : Subsystem
      settings: PortSchema="{\"entries\":[{\"content\":{\"sides\":[{\"content\":{\"connectorIds\":[\"In1\",\"In2\",\"In3\"]},\"type\":\"ConnectorPlacement.EquallySpacedRectSide\",\"uuid\":\"3b61df12-5278-441c-99ea-cd13bbe6a5f0\"},{\"content\":{\"connectorIds\":[\"Out1\"],\"side\":\"RIGHT\"},\"type\":\"ConnectorPlacement.EquallySpacedRectSide\",\"uuid\":\"d74b7cc5-7b27-4e0f-8d84-952eb44d2cfa\"},{\"content\":{\"connectorIds\":[\"Out2\"],\"side\":\"TOP\"},\"type\":\"ConnectorPlacement.EquallySpacedRectSide\",\"uuid\":\"99314f25-b6d9-4ea5-a032-83307ae4bc34\"},{\"content\":{\"connectorIds\":[\"In4\"],\"side\":\"BOTTOM\"},\"type\":\"ConnectorPlacement.EquallySpacedRectSide\",\"uuid\":\"c9c43d88-8d1b-4564-af22-30722c8258ba\"}]},\"type\":\"ConnectorPlacement.EquallySpacedConnector\",\"uuid\":\"25cc7102-d96a-4215-b1b2-f44cf7e448cb\"}],\"packageUris\":[\"http://schema.mathworks.com/mf0/Connector/R2020b\"],\"version\":\"1.0\"}"
  Data Out : Outport
  wires:
  Demux/2 -> Subsystem2/1(A)
  Subtract/1 -> Subsystem/3(Subtract), Subsystem2/3(Subtract), Subsystem3/3(Subtract), Subsystem4/3(Subtract), Subsystem5/3(Subtract), Subsystem6/3(Subtract), Subsystem7/3(Subtract), Subsystem8/3(Subtract), Subsystem1/3(Subtract), Subsystem13/3(Subtract), Subsystem9/3(Subtract), Subsystem10/3(Subtract), Subsystem11/3(Subtract), OR/1
  Subsystem8/2(CO) -> Subsystem7/4(CI)
  Demux/10 -> Subsystem13/1(A)
  Subsystem10/2(CO) -> Subsystem9/4(CI)
  Demux/1 -> Subsystem/1(A)
  Subsystem11/2(CO) -> Subsystem10/4(CI)
  Demux/5 -> Subsystem5/1(A)
  Subsystem10/1(Sum) -> Mux/12  "D4"
  Demux/7 -> Subsystem7/1(A)
  Subsystem3/1(Sum) -> Mux/3  "D4"
  Subsystem6/1(Sum) -> Mux/6  "D4"
  Demux/13 -> Subsystem11/1(A)
  Subsystem5/2(CO) -> Subsystem4/4(CI)
  Demux1/11 -> Subsystem9/2(B)
  OR/1 -> Subsystem11/4(CI)
  Demux1/12 -> Subsystem10/2(B)
  Offset/1 -> Pad/1
  Subsystem2/1(Sum) -> Mux/2  "D4"
  Demux1/9 -> Subsystem1/2(B)
  INC/1 -> OR/2
  Demux1/13 -> Subsystem11/2(B)
  Demux1/8 -> Subsystem8/2(B)
  Demux1/10 -> Subsystem13/2(B)
  Demux1/2 -> Subsystem2/2(B)
  Demux1/1 -> Subsystem/2(B)
  Demux1/6 -> Subsystem6/2(B)
  Subsystem/1(Sum) -> Mux/1  "D4"
  Demux1/3 -> Subsystem3/2(B)
  Demux1/7 -> Subsystem7/2(B)
  Demux1/4 -> Subsystem4/2(B)
  Subsystem4/2(CO) -> Subsystem3/4(CI)
  Subsystem7/1(Sum) -> Mux/7  "D4"
  Demux/6 -> Subsystem6/1(A)
  Subsystem6/2(CO) -> Subsystem5/4(CI)
  Demux1/5 -> Subsystem5/2(B)
  Subsystem7/2(CO) -> Subsystem6/4(CI)
  Subsystem3/2(CO) -> Subsystem2/4(CI)
  Subsystem5/1(Sum) -> Mux/5  "D4"
  Subsystem2/2(CO) -> Subsystem/4(CI)
  Subsystem1/1(Sum) -> Mux/9  "D4"
  Subsystem8/1(Sum) -> Mux/8  "D4"
  Subsystem11/1(Sum) -> Mux/13  "D4"
  Subsystem13/2(CO) -> Subsystem1/4(CI)
  Subsystem9/1(Sum) -> Mux/11  "D4"
  Subsystem1/2(CO) -> Subsystem8/4(CI)
  Demux/9 -> Subsystem1/1(A)
  Demux/11 -> Subsystem9/1(A)
  Mux/1 -> Data Out/1
  Subsystem9/2(CO) -> Subsystem13/4(CI)
  Subsystem13/1(Sum) -> Mux/10  "D4"
  Demux/8 -> Subsystem8/1(A)
  Demux/4 -> Subsystem4/1(A)
  Data In/1 -> Demux/1
  Subsystem4/1(Sum) -> Mux/4  "D4"
  Demux/3 -> Subsystem3/1(A)
  Demux/12 -> Subsystem10/1(A)
  Pad/1 -> Demux1/1
